simulink model "gm_HA_sys8_vnl"  (R2018a)
settings: Solver=FixedStepDiscrete  StartTime=0.0  StopTime=stopTime  RelTol=1e-3
InitFcn:
  | HA_sys8_init
StopFcn:
  | HA_sys8_freq_response
undefined symbols (not defined in the file or in its folder): dspDeleteFVToolLinkFromMask, FIRBandPass1, FIRBandPass2, FIRBandPass3, FIRBandPass4, FIRDecimator1, FIRDecimator2, FIRDecimator3, FIRDecimator4, FIRInterpolator1, FIRInterpolator2, FIRInterpolator3, FIRInterpolator4, Fs, Gain_B1_left, Gain_B1_right, Gain_B2_left, Gain_B2_right, Gain_B3_left, Gain_B3_right, Gain_B4_left, Gain_B4_right, Gain_left_all, Gain_right_all, gcbh
libraries: hdlsllib x40, dspmlti4 x32, simulink x4, dspsrcs4 x1
(part 1 of 4)
settings Model: Creator=The MathWorks, Inc.  LastModifiedBy=Ross_admin
settings DataIOCC: LimitDataPoints=on  SaveFormat=Array  SaveOutput=off  SaveTime=off
settings OptimizationCC: BlockReduction=off  ConditionallyExecuteInputs=off  DefaultParameterBehavior=Inlined  LifeSpan=inf
settings DebuggingCC: AlgebraicLoopMsg=error  InheritedTsInSrcMsg=none  SingleTaskRateTransMsg=error  AllowSymbolicDim=off  StrictBusMsg=ErrorOnBusTreatedAsVector  SFUnexpectedBacktrackingDiag=warning  SFNoUnconditionalDefaultTransitionDiag=warning  SFExecutionAtInitializationDiag=none
settings HardwareCC: ProdBitPerPointer=32  ProdBitPerSizeT=32  ProdBitPerPtrDiffT=32  ProdLargestAtomicFloat=None  ProdIntDivRoundTo=Undefined  ProdEndianess=Unspecified  ProdWordSize=32  ProdHWDeviceType=ASIC/FPGA->ASIC/FPGA  ProdEqTarget=off
settings ModelReferenceCC: PropagateSignalLabelsOutOfModel=off
settings CodeAppCC: StateflowObjectComments=on
settings GRTTargetCC: TargetLangStandard=C89/C90 (ANSI)  GeneratePreprocessorConditionals=Disable all
settings ConfigComp: CovMetricSettings=dw  CovHtmlReporting=on  CovSaveCumulativeToWorkspaceVar=on  CovSaveSingleToWorkspaceVar=on  CovShowResultsExplorer=off  CovExternalEMLEnable=off

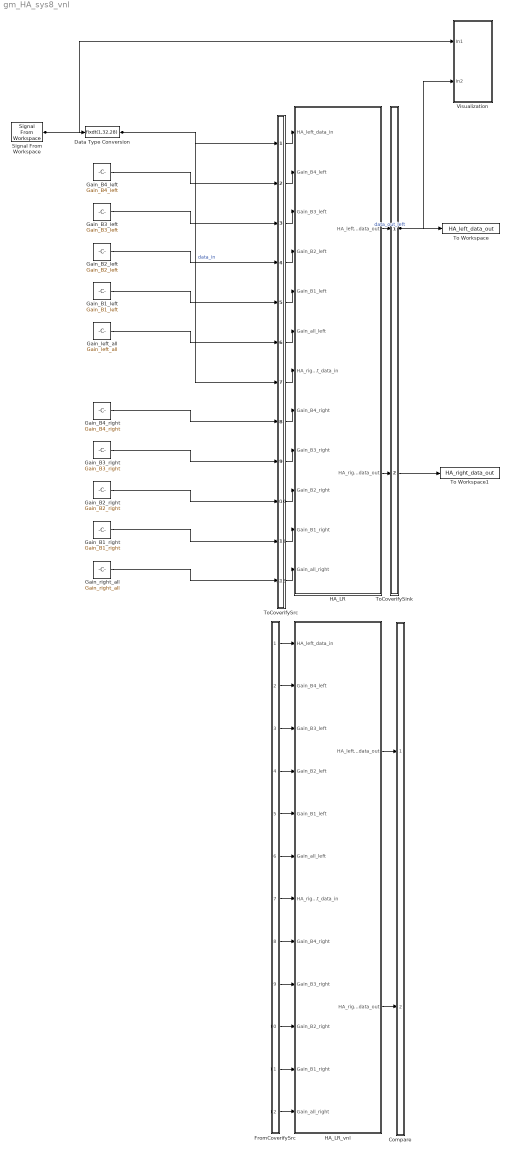
== system gm_HA_sys8_vnl ==
  Compare : Subsystem
      mask Display: disp('')
  Data Type Conversion : DataTypeConversion  OutDataTypeStr=fixdt(1,32,28)
  FromCoverifySrc : Subsystem
      mask Display: disp('')
  Gain_B1_left : Constant  Value=Gain_B1_left  OutDataTypeStr=fixdt(1,32,16)  SampleTime=-1  LockScale=on
  Gain_B1_right : Constant  Value=Gain_B1_right  OutDataTypeStr=fixdt(1,32,16)  SampleTime=-1  LockScale=on
  Gain_B2_left : Constant  Value=Gain_B2_left  OutDataTypeStr=fixdt(1,32,16)  SampleTime=-1  LockScale=on
  Gain_B2_right : Constant  Value=Gain_B2_right  OutDataTypeStr=fixdt(1,32,16)  SampleTime=-1  LockScale=on
  Gain_B3_left : Constant  Value=Gain_B3_left  OutDataTypeStr=fixdt(1,32,16)  SampleTime=-1  LockScale=on
  Gain_B3_right : Constant  Value=Gain_B3_right  OutDataTypeStr=fixdt(1,32,16)  SampleTime=-1  LockScale=on
  Gain_B4_left : Constant  Value=Gain_B4_left  OutDataTypeStr=fixdt(1,32,16)  SampleTime=-1  LockScale=on
  Gain_B4_right : Constant  Value=Gain_B4_right  OutDataTypeStr=fixdt(1,32,16)  SampleTime=-1  LockScale=on
  Gain_left_all : Constant  Value=Gain_left_all  OutDataTypeStr=fixdt(1,32,16)  SampleTime=-1  LockScale=on
  Gain_right_all : Constant  Value=Gain_right_all  OutDataTypeStr=fixdt(1,32,16)  SampleTime=-1  LockScale=on
  HA_LR : Subsystem
  HA_LR_vnl : Subsystem
  Signal From Workspace : dspsrcs4/Signal From Workspace  X=signal_in  Ts=1/Fs  nsamps=1  OutputAfterFinalValue=Setting to zero  ignoreOrWarnInputAndFrameLengths=off  OutputFrames=off
  To Workspace : ToWorkspace  VariableName=HA_left_data_out  SampleTime=-1
      settings: Save2DSignal=2-D array (concatenate along first dimension)
  To Workspace1 : ToWorkspace  VariableName=HA_right_data_out  SampleTime=-1
      settings: Save2DSignal=2-D array (concatenate along first dimension)
  ToCoverifySink : Subsystem
      mask Display: disp('')
  ToCoverifySrc : Subsystem
      mask Display: disp('')
  Visualization : Subsystem
      mask Display: disp('SCOPES')
  wires:
  Signal From Workspace/1 -> Visualization/1(In1), Data Type Conversion/1
  ToCoverifySrc/1(out1) -> HA_LR/1(HA_left_data_in)
  ToCoverifySrc/2(out2) -> HA_LR/2(Gain_B4_left)
  ToCoverifySrc/3(out3) -> HA_LR/3(Gain_B3_left)
  ToCoverifySrc/4(out4) -> HA_LR/4(Gain_B2_left)
  ToCoverifySrc/5(out5) -> HA_LR/5(Gain_B1_left)
  ToCoverifySrc/6(out6) -> HA_LR/6(Gain_all_left)
  ToCoverifySrc/7(out7) -> HA_LR/7(HA_right_data_in)
  ToCoverifySrc/8(out8) -> HA_LR/8(Gain_B4_right)
  ToCoverifySrc/9(out9) -> HA_LR/9(Gain_B3_right)
  ToCoverifySrc/10(out10) -> HA_LR/10(Gain_B2_right)
  ToCoverifySrc/11(out11) -> HA_LR/11(Gain_B1_right)
  ToCoverifySrc/12(out12) -> HA_LR/12(Gain_all_right)
  HA_LR/1(HA_left_data_out) -> ToCoverifySink/1(in1)  "data_out_left"
  HA_LR/2(HA_right_data_out) -> ToCoverifySink/2(in2)
  Data Type Conversion/1 -> ToCoverifySrc/1(in1), ToCoverifySrc/7(in7)  "data_in"
  Gain_B4_left/1 -> ToCoverifySrc/2(in2)
  Gain_B3_left/1 -> ToCoverifySrc/3(in3)
  Gain_B2_left/1 -> ToCoverifySrc/4(in4)
  Gain_B1_left/1 -> ToCoverifySrc/5(in5)
  Gain_left_all/1 -> ToCoverifySrc/6(in6)
  Gain_B4_right/1 -> ToCoverifySrc/8(in8)
  Gain_B3_right/1 -> ToCoverifySrc/9(in9)
  Gain_B2_right/1 -> ToCoverifySrc/10(in10)
  Gain_B1_right/1 -> ToCoverifySrc/11(in11)
  Gain_right_all/1 -> ToCoverifySrc/12(in12)
  ToCoverifySink/1(out1) -> To Workspace/1, Visualization/2(In2)
  ToCoverifySink/2(out2) -> To Workspace1/1
  FromCoverifySrc/1(out1) -> HA_LR_vnl/1(HA_left_data_in)
  FromCoverifySrc/2(out2) -> HA_LR_vnl/2(Gain_B4_left)
  FromCoverifySrc/3(out3) -> HA_LR_vnl/3(Gain_B3_left)
  FromCoverifySrc/4(out4) -> HA_LR_vnl/4(Gain_B2_left)
  FromCoverifySrc/5(out5) -> HA_LR_vnl/5(Gain_B1_left)
  FromCoverifySrc/6(out6) -> HA_LR_vnl/6(Gain_all_left)
  FromCoverifySrc/7(out7) -> HA_LR_vnl/7(HA_right_data_in)
  FromCoverifySrc/8(out8) -> HA_LR_vnl/8(Gain_B4_right)
  FromCoverifySrc/9(out9) -> HA_LR_vnl/9(Gain_B3_right)
  FromCoverifySrc/10(out10) -> HA_LR_vnl/10(Gain_B2_right)
  FromCoverifySrc/11(out11) -> HA_LR_vnl/11(Gain_B1_right)
  FromCoverifySrc/12(out12) -> HA_LR_vnl/12(Gain_all_right)
  HA_LR_vnl/1(HA_left_data_out) -> Compare/1(in1)
  HA_LR_vnl/2(HA_right_data_out) -> Compare/2(in2)

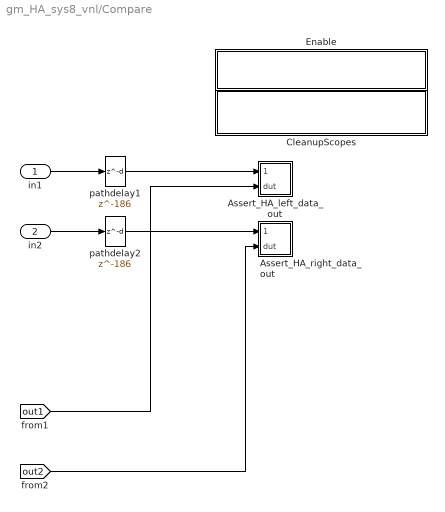
== system gm_HA_sys8_vnl/Compare ==
  in1 : Inport
  in2 : Inport  Port=2
  Assert_HA_left_data_out : Subsystem
  Assert_HA_right_data_out : Subsystem
  CleanupScopes : Subsystem
      settings: OpenFcn=|
      | blkName = gcb; %self block
      | idx = regexp(blkName, '/CleanupScopes$', 'once');
      | blkParent = blkName(1:idx-1);
      | blks=find_system(blkParent, 'LookUnderMasks', 'all','blocktype', 'Scope');
      | for itr = 1:length(blks)
      | 	 hScopeCfg = get_param(blks{itr},'ScopeConfiguration');
      | 	 hScopeCfg.Visible = ~ hScopeCfg.Visible;
      | end
      | drawnow;
      mask Display: fprintf(message('hdlcoder:cosim:vnl_dblclick').getString());
  Enable : Subsystem
      settings: OpenFcn=|
      | blkName = gcb;
      | idx = regexp(blkName, '/Enable$', 'once');
      | blkParent = blkName(1:idx-1);
      | blks=find_system(blkParent, 'LookUnderMasks', 'all','blocktype', 'Assertion');
      | e = get_param(blks{1}, 'Enabled');
      | if strcmp(e, 'on'), f= 'off';, else, f = 'on';, end
      | for ii=1:length(blks), set_param(blks{ii}, 'Enabled', f);, end
      | set_param(gcb, 'MaskDisplay',['fprintf(message(''hdlcoder:cosim:vnl_dblclick_assertions'',','''',upper(e),'''',').getString())']);
      mask Display: fprintf(message('hdlcoder:cosim:vnl_dblclick_assertions','OFF').getString());
  pathdelay1 : Delay  DelayLength=186
  pathdelay2 : Delay  DelayLength=186
  wires:
  in1/1 -> pathdelay1/1
  pathdelay1/1 -> Assert_HA_left_data_out/1(cosim)
  [out1] -> Assert_HA_left_data_out/2(dut)
  in2/1 -> pathdelay2/1
  pathdelay2/1 -> Assert_HA_right_data_out/1(cosim)
  [out2] -> Assert_HA_right_data_out/2(dut)

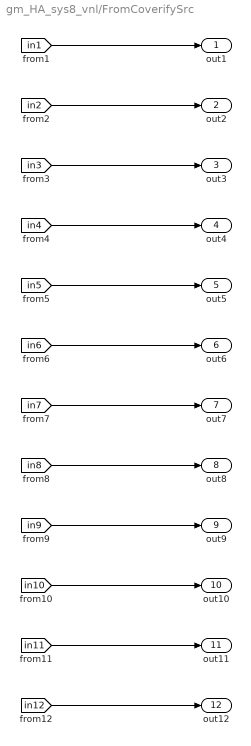
== system gm_HA_sys8_vnl/FromCoverifySrc ==
  out1 : Outport
  out2 : Outport  Port=2
  out3 : Outport  Port=3
  out4 : Outport  Port=4
  out5 : Outport  Port=5
  out6 : Outport  Port=6
  out7 : Outport  Port=7
  out8 : Outport  Port=8
  out9 : Outport  Port=9
  out10 : Outport  Port=10
  out11 : Outport  Port=11
  out12 : Outport  Port=12
  wires:
  [in1] -> out1/1
  [in2] -> out2/1
  [in3] -> out3/1
  [in4] -> out4/1
  [in5] -> out5/1
  [in6] -> out6/1
  [in7] -> out7/1
  [in8] -> out8/1
  [in9] -> out9/1
  [in10] -> out10/1
  [in11] -> out11/1
  [in12] -> out12/1

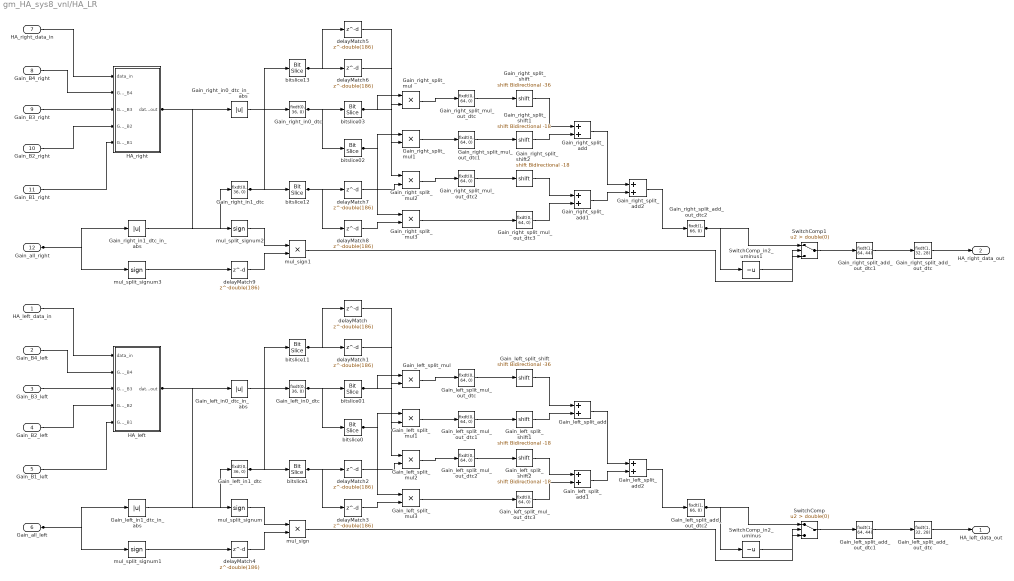
== system gm_HA_sys8_vnl/HA_LR ==
  HA_left_data_in : Inport  OutDataTypeStr=fixdt(1, 32, 28)  PortDimensions=1  SampleTime=2.08333333333333e-05
  Gain_B4_left : Inport  Port=2  OutDataTypeStr=fixdt(1, 32, 16)  PortDimensions=1  SampleTime=8.33333333333333e-05
  Gain_B3_left : Inport  Port=3  OutDataTypeStr=fixdt(1, 32, 16)  PortDimensions=1  SampleTime=0.000166666666666667
  Gain_B2_left : Inport  Port=4  OutDataTypeStr=fixdt(1, 32, 16)  PortDimensions=1  SampleTime=0.000333333333333333
  Gain_B1_left : Inport  Port=5  OutDataTypeStr=fixdt(1, 32, 16)  PortDimensions=1  SampleTime=0.000666666666666667
  Gain_all_left : Inport  Port=6  OutDataTypeStr=fixdt(1, 32, 16)  PortDimensions=1  SampleTime=2.08333333333333e-05
  HA_right_data_in : Inport  Port=7  OutDataTypeStr=fixdt(1, 32, 28)  PortDimensions=1  SampleTime=2.08333333333333e-05
  Gain_B4_right : Inport  Port=8  OutDataTypeStr=fixdt(1, 32, 16)  PortDimensions=1  SampleTime=8.33333333333333e-05
  Gain_B3_right : Inport  Port=9  OutDataTypeStr=fixdt(1, 32, 16)  PortDimensions=1  SampleTime=0.000166666666666667
  Gain_B2_right : Inport  Port=10  OutDataTypeStr=fixdt(1, 32, 16)  PortDimensions=1  SampleTime=0.000333333333333333
  Gain_B1_right : Inport  Port=11  OutDataTypeStr=fixdt(1, 32, 16)  PortDimensions=1  SampleTime=0.000666666666666667
  Gain_all_right : Inport  Port=12  OutDataTypeStr=fixdt(1, 32, 16)  PortDimensions=1  SampleTime=2.08333333333333e-05
  Gain_left_in0_dtc : DataTypeConversion  OutDataTypeStr=fixdt(0, 36, 0)  ConvertRealWorld=Stored Integer (SI)  SampleTime=2.08333333333333e-05
  Gain_left_in0_dtc_in_abs : Abs  SampleTime=2.08333333333333e-05  OutDataTypeStr=fixdt(0, 32, 28)
  Gain_left_in1_dtc : DataTypeConversion  OutDataTypeStr=fixdt(0, 36, 0)  ConvertRealWorld=Stored Integer (SI)  SampleTime=2.08333333333333e-05
  Gain_left_in1_dtc_in_abs : Abs  SampleTime=2.08333333333333e-05  OutDataTypeStr=fixdt(0, 32, 16)
  Gain_left_split_add : Sum  OutDataTypeStr=fixdt(0, 65, 0)  SampleTime=2.08333333333333e-05
  Gain_left_split_add1 : Sum  OutDataTypeStr=fixdt(0, 65, 0)  SampleTime=2.08333333333333e-05
  Gain_left_split_add2 : Sum  OutDataTypeStr=fixdt(0, 66, 0)  SampleTime=2.08333333333333e-05
  Gain_left_split_add_out_dtc : DataTypeConversion  OutDataTypeStr=fixdt(1, 32, 28)  SampleTime=2.08333333333333e-05  SaturateOnIntegerOverflow=on
  Gain_left_split_add_out_dtc1 : DataTypeConversion  OutDataTypeStr=fixdt(1, 64, 44)  ConvertRealWorld=Stored Integer (SI)  SampleTime=2.08333333333333e-05
  Gain_left_split_add_out_dtc2 : DataTypeConversion  OutDataTypeStr=fixdt(1, 66, 0)  SampleTime=2.08333333333333e-05
  Gain_left_split_mul : Product  Inputs=**  OutDataTypeStr=fixdt(0, 28, 0)  SampleTime=2.08333333333333e-05
  Gain_left_split_mul1 : Product  Inputs=**  OutDataTypeStr=uint32  SampleTime=2.08333333333333e-05
  Gain_left_split_mul2 : Product  Inputs=**  OutDataTypeStr=uint32  SampleTime=2.08333333333333e-05
  Gain_left_split_mul3 : Product  Inputs=**  OutDataTypeStr=fixdt(0, 36, 0)  SampleTime=2.08333333333333e-05
  Gain_left_split_mul_out_dtc{,1..3} (4 alike) : DataTypeConversion  OutDataTypeStr=fixdt(0, 64, 0)  SampleTime=2.08333333333333e-05
  Gain_left_split_shift : ArithShift  BitShiftNumber=-36
  Gain_left_split_shift1 : ArithShift  BitShiftNumber=-18
  Gain_left_split_shift2 : ArithShift  BitShiftNumber=-18
  Gain_right_in0_dtc : DataTypeConversion  OutDataTypeStr=fixdt(0, 36, 0)  ConvertRealWorld=Stored Integer (SI)  SampleTime=2.08333333333333e-05
  Gain_right_in0_dtc_in_abs : Abs  SampleTime=2.08333333333333e-05  OutDataTypeStr=fixdt(0, 32, 28)
  Gain_right_in1_dtc : DataTypeConversion  OutDataTypeStr=fixdt(0, 36, 0)  ConvertRealWorld=Stored Integer (SI)  SampleTime=2.08333333333333e-05
  Gain_right_in1_dtc_in_abs : Abs  SampleTime=2.08333333333333e-05  OutDataTypeStr=fixdt(0, 32, 16)
  Gain_right_split_add : Sum  OutDataTypeStr=fixdt(0, 65, 0)  SampleTime=2.08333333333333e-05
  Gain_right_split_add1 : Sum  OutDataTypeStr=fixdt(0, 65, 0)  SampleTime=2.08333333333333e-05
  Gain_right_split_add2 : Sum  OutDataTypeStr=fixdt(0, 66, 0)  SampleTime=2.08333333333333e-05
  Gain_right_split_add_out_dtc : DataTypeConversion  OutDataTypeStr=fixdt(1, 32, 28)  SampleTime=2.08333333333333e-05  SaturateOnIntegerOverflow=on
  Gain_right_split_add_out_dtc1 : DataTypeConversion  OutDataTypeStr=fixdt(1, 64, 44)  ConvertRealWorld=Stored Integer (SI)  SampleTime=2.08333333333333e-05
  Gain_right_split_add_out_dtc2 : DataTypeConversion  OutDataTypeStr=fixdt(1, 66, 0)  SampleTime=2.08333333333333e-05
  Gain_right_split_mul : Product  Inputs=**  OutDataTypeStr=fixdt(0, 28, 0)  SampleTime=2.08333333333333e-05
  Gain_right_split_mul1 : Product  Inputs=**  OutDataTypeStr=uint32  SampleTime=2.08333333333333e-05
  Gain_right_split_mul2 : Product  Inputs=**  OutDataTypeStr=uint32  SampleTime=2.08333333333333e-05
  Gain_right_split_mul3 : Product  Inputs=**  OutDataTypeStr=fixdt(0, 36, 0)  SampleTime=2.08333333333333e-05
  Gain_right_split_mul_out_dtc{,1..3} (4 alike) : DataTypeConversion  OutDataTypeStr=fixdt(0, 64, 0)  SampleTime=2.08333333333333e-05
  Gain_right_split_shift : ArithShift  BitShiftNumber=-36
  Gain_right_split_shift1 : ArithShift  BitShiftNumber=-18
  Gain_right_split_shift2 : ArithShift  BitShiftNumber=-18
  HA_left : Subsystem
  HA_right : Subsystem
  SwitchComp : Switch  Criteria=u2 > Threshold  Threshold=double(0)  OutDataTypeStr=fixdt(1, 66, 0)  SampleTime=2.08333333333333e-05
  SwitchComp1 : Switch  Criteria=u2 > Threshold  Threshold=double(0)  OutDataTypeStr=fixdt(1, 66, 0)  SampleTime=2.08333333333333e-05
  SwitchComp_in2_uminus : UnaryMinus  SampleTime=2.08333333333333e-05
  SwitchComp_in2_uminus1 : UnaryMinus  SampleTime=2.08333333333333e-05
  bitslice0 : hdlsllib/Logic and Bit Operations/Bit Slice  lidx=double(17)  ridx=double(0)
  bitslice01 : hdlsllib/Logic and Bit Operations/Bit Slice  lidx=double(31)  ridx=double(18)
  bitslice02 : hdlsllib/Logic and Bit Operations/Bit Slice  lidx=double(17)  ridx=double(0)
  bitslice03 : hdlsllib/Logic and Bit Operations/Bit Slice  lidx=double(31)  ridx=double(18)
  bitslice1 : hdlsllib/Logic and Bit Operations/Bit Slice  lidx=double(17)  ridx=double(0)
  bitslice11 : hdlsllib/Logic and Bit Operations/Bit Slice  lidx=double(31)  ridx=double(18)
  bitslice12 : hdlsllib/Logic and Bit Operations/Bit Slice  lidx=double(17)  ridx=double(0)
  bitslice13 : hdlsllib/Logic and Bit Operations/Bit Slice  lidx=double(31)  ridx=double(18)
  delayMatch{,1..9} (10 alike) : Delay  DelayLength=double(186)  InitialCondition=0  InputProcessing=Inherited  SampleTime=2.08333333333333e-05
  mul_sign : Product  Inputs=**  OutDataTypeStr=fixdt(1, 2, 0)  SampleTime=2.08333333333333e-05
  mul_sign1 : Product  Inputs=**  OutDataTypeStr=fixdt(1, 2, 0)  SampleTime=2.08333333333333e-05
  mul_split_signum{,1..3} (4 alike) : Signum  SampleTime=2.08333333333333e-05
  HA_left_data_out : Outport
  HA_right_data_out : Outport  Port=2
  wires:
  mul_split_signum3/1 -> delayMatch9/1
  bitslice12/1 -> delayMatch7/1, delayMatch8/1
  delayMatch8/1 -> Gain_right_split_mul3/2
  bitslice13/1 -> delayMatch5/1, delayMatch6/1
  delayMatch6/1 -> Gain_right_split_mul1/2
  mul_split_signum1/1 -> delayMatch4/1
  bitslice1/1 -> delayMatch2/1, delayMatch3/1
  delayMatch3/1 -> Gain_left_split_mul3/2
  bitslice11/1 -> delayMatch/1, delayMatch1/1
  delayMatch1/1 -> Gain_left_split_mul1/2
  SwitchComp_in2_uminus1/1 -> SwitchComp1/3
  SwitchComp1/1 -> Gain_right_split_add_out_dtc1/1
  Gain_right_split_add2/1 -> Gain_right_split_add_out_dtc2/1
  mul_sign1/1 -> SwitchComp1/2
  delayMatch9/1 -> mul_sign1/2
  Gain_right_in1_dtc_in_abs/1 -> Gain_right_in1_dtc/1
  mul_split_signum2/1 -> mul_sign1/1
  Gain_right_in0_dtc_in_abs/1 -> Gain_right_in0_dtc/1
  Gain_right_split_add_out_dtc2/1 -> SwitchComp1/1, SwitchComp_in2_uminus1/1
  Gain_right_split_add_out_dtc1/1 -> Gain_right_split_add_out_dtc/1
  Gain_right_split_add_out_dtc/1 -> HA_right_data_out/1
  Gain_right_split_add1/1 -> Gain_right_split_add2/2
  Gain_right_split_add/1 -> Gain_right_split_add2/1
  Gain_right_split_mul3/1 -> Gain_right_split_mul_out_dtc3/1
  Gain_right_split_mul_out_dtc3/1 -> Gain_right_split_add1/2
  Gain_right_split_shift2/1 -> Gain_right_split_add1/1
  Gain_right_split_mul2/1 -> Gain_right_split_mul_out_dtc2/1
  Gain_right_split_mul_out_dtc2/1 -> Gain_right_split_shift2/1
  Gain_right_split_shift1/1 -> Gain_right_split_add/2
  Gain_right_split_mul1/1 -> Gain_right_split_mul_out_dtc1/1
  Gain_right_split_mul_out_dtc1/1 -> Gain_right_split_shift1/1
  Gain_right_split_shift/1 -> Gain_right_split_add/1
  Gain_right_split_mul/1 -> Gain_right_split_mul_out_dtc/1
  Gain_right_split_mul_out_dtc/1 -> Gain_right_split_shift/1
  delayMatch5/1 -> Gain_right_split_mul/2
  delayMatch7/1 -> Gain_right_split_mul2/2
  bitslice03/1 -> Gain_right_split_mul/1, Gain_right_split_mul2/1
  bitslice02/1 -> Gain_right_split_mul1/1, Gain_right_split_mul3/1
  Gain_right_in1_dtc/1 -> bitslice12/1, bitslice13/1
  Gain_right_in0_dtc/1 -> bitslice02/1, bitslice03/1
  SwitchComp_in2_uminus/1 -> SwitchComp/3
  SwitchComp/1 -> Gain_left_split_add_out_dtc1/1
  Gain_left_split_add2/1 -> Gain_left_split_add_out_dtc2/1
  mul_sign/1 -> SwitchComp/2
  delayMatch4/1 -> mul_sign/2
  Gain_left_in1_dtc_in_abs/1 -> Gain_left_in1_dtc/1
  mul_split_signum/1 -> mul_sign/1
  Gain_left_in0_dtc_in_abs/1 -> Gain_left_in0_dtc/1
  Gain_left_split_add_out_dtc2/1 -> SwitchComp/1, SwitchComp_in2_uminus/1
  Gain_left_split_add_out_dtc1/1 -> Gain_left_split_add_out_dtc/1
  Gain_left_split_add_out_dtc/1 -> HA_left_data_out/1
  Gain_left_split_add1/1 -> Gain_left_split_add2/2
  Gain_left_split_add/1 -> Gain_left_split_add2/1
  Gain_left_split_mul3/1 -> Gain_left_split_mul_out_dtc3/1
  Gain_left_split_mul_out_dtc3/1 -> Gain_left_split_add1/2
  Gain_left_split_shift2/1 -> Gain_left_split_add1/1
  Gain_left_split_mul2/1 -> Gain_left_split_mul_out_dtc2/1
  Gain_left_split_mul_out_dtc2/1 -> Gain_left_split_shift2/1
  Gain_left_split_shift1/1 -> Gain_left_split_add/2
  Gain_left_split_mul1/1 -> Gain_left_split_mul_out_dtc1/1
  Gain_left_split_mul_out_dtc1/1 -> Gain_left_split_shift1/1
  Gain_left_split_shift/1 -> Gain_left_split_add/1
  Gain_left_split_mul/1 -> Gain_left_split_mul_out_dtc/1
  Gain_left_split_mul_out_dtc/1 -> Gain_left_split_shift/1
  delayMatch/1 -> Gain_left_split_mul/2
  delayMatch2/1 -> Gain_left_split_mul2/2
  bitslice01/1 -> Gain_left_split_mul/1, Gain_left_split_mul2/1
  bitslice0/1 -> Gain_left_split_mul1/1, Gain_left_split_mul3/1
  Gain_left_in1_dtc/1 -> bitslice1/1, bitslice11/1
  Gain_left_in0_dtc/1 -> bitslice0/1, bitslice01/1
  HA_right/1(data_out) -> Gain_right_in0_dtc_in_abs/1, mul_split_signum2/1
  HA_left/1(data_out) -> Gain_left_in0_dtc_in_abs/1, mul_split_signum/1
  Gain_all_right/1 -> Gain_right_in1_dtc_in_abs/1, mul_split_signum3/1
  Gain_B1_right/1 -> HA_right/5(Gain_B1)
  Gain_B2_right/1 -> HA_right/4(Gain_B2)
  Gain_B3_right/1 -> HA_right/3(Gain_B3)
  Gain_B4_right/1 -> HA_right/2(Gain_B4)
  HA_right_data_in/1 -> HA_right/1(data_in)
  Gain_all_left/1 -> Gain_left_in1_dtc_in_abs/1, mul_split_signum1/1
  Gain_B1_left/1 -> HA_left/5(Gain_B1)
  Gain_B2_left/1 -> HA_left/4(Gain_B2)
  Gain_B3_left/1 -> HA_left/3(Gain_B3)
  Gain_B4_left/1 -> HA_left/2(Gain_B4)
  HA_left_data_in/1 -> HA_left/1(data_in)

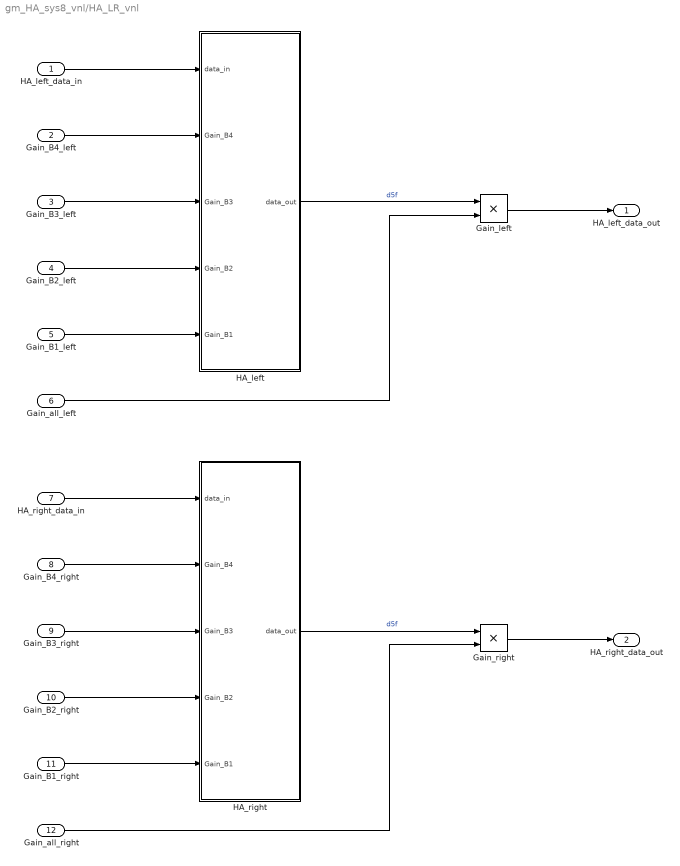
== system gm_HA_sys8_vnl/HA_LR_vnl ==
  HA_left_data_in : Inport
  Gain_B4_left : Inport  Port=2
  Gain_B3_left : Inport  Port=3
  Gain_B2_left : Inport  Port=4
  Gain_B1_left : Inport  Port=5
  Gain_all_left : Inport  Port=6
  HA_right_data_in : Inport  Port=7
  Gain_B4_right : Inport  Port=8
  Gain_B3_right : Inport  Port=9
  Gain_B2_right : Inport  Port=10
  Gain_B1_right : Inport  Port=11
  Gain_all_right : Inport  Port=12
  Gain_left : Product  OutDataTypeStr=fixdt(1,32,28)  SaturateOnIntegerOverflow=on
  Gain_right : Product  OutDataTypeStr=fixdt(1,32,28)  SaturateOnIntegerOverflow=on
  HA_left : Subsystem
  HA_right : Subsystem
  HA_left_data_out : Outport
  HA_right_data_out : Outport  Port=2
  wires:
  HA_right/1(data_out) -> Gain_right/1  "d5f"
  Gain_all_right/1 -> Gain_right/2
  HA_right_data_in/1 -> HA_right/1(data_in)
  Gain_B3_right/1 -> HA_right/3(Gain_B3)
  Gain_B2_right/1 -> HA_right/4(Gain_B2)
  Gain_right/1 -> HA_right_data_out/1
  Gain_B4_right/1 -> HA_right/2(Gain_B4)
  Gain_B1_right/1 -> HA_right/5(Gain_B1)
  Gain_left/1 -> HA_left_data_out/1
  Gain_all_left/1 -> Gain_left/2
  HA_left/1(data_out) -> Gain_left/1  "d5f"
  Gain_B4_left/1 -> HA_left/2(Gain_B4)
  HA_left_data_in/1 -> HA_left/1(data_in)
  Gain_B2_left/1 -> HA_left/4(Gain_B2)
  Gain_B3_left/1 -> HA_left/3(Gain_B3)
  Gain_B1_left/1 -> HA_left/5(Gain_B1)

== system gm_HA_sys8_vnl/ToCoverifySink ==
  in1 : Inport
  in2 : Inport  Port=2
  out1 : Outport
  out2 : Outport  Port=2
  tag scope: out1=global, out2=global
  wires:
  in1/1 -> out1/1, [out1]
  in2/1 -> out2/1, [out2]

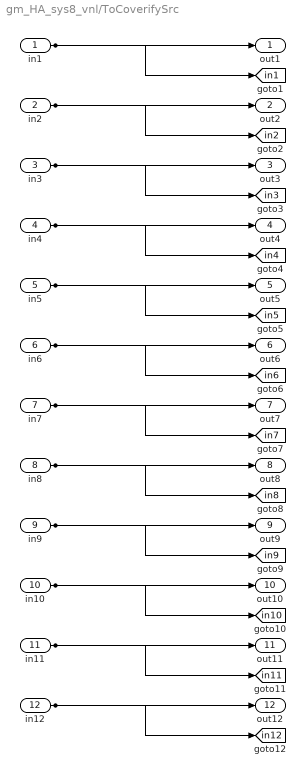
== system gm_HA_sys8_vnl/ToCoverifySrc ==
  in1 : Inport
  in2 : Inport  Port=2
  in3 : Inport  Port=3
  in4 : Inport  Port=4
  in5 : Inport  Port=5
  in6 : Inport  Port=6
  in7 : Inport  Port=7
  in8 : Inport  Port=8
  in9 : Inport  Port=9
  in10 : Inport  Port=10
  in11 : Inport  Port=11
  in12 : Inport  Port=12
  out1 : Outport
  out2 : Outport  Port=2
  out3 : Outport  Port=3
  out4 : Outport  Port=4
  out5 : Outport  Port=5
  out6 : Outport  Port=6
  out7 : Outport  Port=7
  out8 : Outport  Port=8
  out9 : Outport  Port=9
  out10 : Outport  Port=10
  out11 : Outport  Port=11
  out12 : Outport  Port=12
  tag scope: in10=global, in11=global, in12=global, in1=global, in2=global, in3=global, in4=global, in5=global, in6=global, in7=global, in8=global, in9=global
  wires:
  in1/1 -> out1/1, [in1]
  in2/1 -> out2/1, [in2]
  in3/1 -> out3/1, [in3]
  in4/1 -> out4/1, [in4]
  in5/1 -> out5/1, [in5]
  in6/1 -> out6/1, [in6]
  in7/1 -> out7/1, [in7]
  in8/1 -> out8/1, [in8]
  in9/1 -> out9/1, [in9]
  in10/1 -> out10/1, [in10]
  in11/1 -> out11/1, [in11]
  in12/1 -> out12/1, [in12]

== system gm_HA_sys8_vnl/Visualization ==
  In1 : Inport
  In2 : Inport  Port=2
  Input Signal (dB Magnitude) : Scope
  Input Signal Spectrum : SpectrumAnalyzer
  Output Signal (dB Mag - passband scale) : Scope
  Output Signal Spectrum : SpectrumAnalyzer
  wires:
  In1/1 -> Input Signal Spectrum/1, Input Signal (dB Magnitude)/1
  In2/1 -> Output Signal Spectrum/1, Output Signal (dB Mag - passband scale)/1

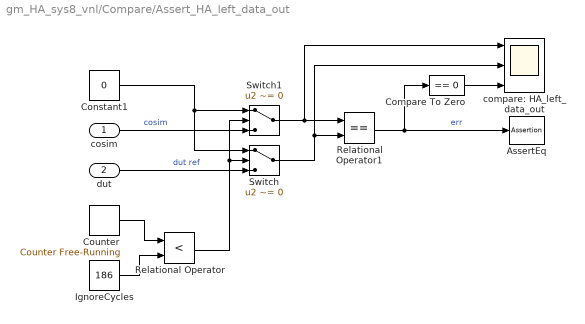
== system gm_HA_sys8_vnl/Compare/Assert_HA_left_data_out ==
  cosim : Inport
  dut : Inport  Port=2
  AssertEq : Assertion  StopWhenAssertionFail=off
  Compare To Zero : simulink/Logic and Bit Operations/Compare To Zero  relop===  OutDataTypeStr=boolean
  Constant1 : Constant  Value=0  OutDataTypeStr=Inherit: Inherit via back propagation  SampleTime=-1
  Counter : simulink/Sources/Counter Free-Running  NumBits=32  tsamp=-1
  IgnoreCycles : Constant  Value=186  OutDataTypeStr=Inherit: Inherit via back propagation  SampleTime=-1
  Relational Operator : RelationalOperator  Operator=<  OutDataTypeStr=boolean  RndMeth=Nearest
  Relational Operator1 : RelationalOperator  Operator===  OutDataTypeStr=boolean  RndMeth=Nearest
  Switch : Switch  Criteria=u2 ~= 0
  Switch1 : Switch  Criteria=u2 ~= 0
  compare: HA_left_data_out : Scope  NumInputPorts=3
  wires:
  Compare To Zero/1 -> compare: HA_left_data_out/3
  Relational Operator1/1 -> Compare To Zero/1, AssertEq/1  "err"
  Switch1/1 -> compare: HA_left_data_out/1, Relational Operator1/1
  Switch/1 -> compare: HA_left_data_out/2, Relational Operator1/2
  Constant1/1 -> Switch/1, Switch1/1
  Relational Operator/1 -> Switch/2, Switch1/2
  cosim/1 -> Switch1/3  "cosim"
  dut/1 -> Switch/3  "dut ref"
  Counter/1 -> Relational Operator/1
  IgnoreCycles/1 -> Relational Operator/2

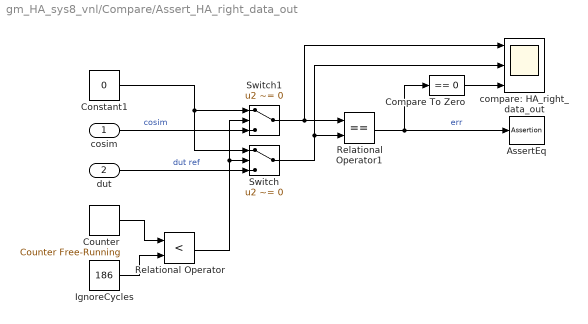
== system gm_HA_sys8_vnl/Compare/Assert_HA_right_data_out ==
  cosim : Inport
  dut : Inport  Port=2
  AssertEq : Assertion  StopWhenAssertionFail=off
  Compare To Zero : simulink/Logic and Bit Operations/Compare To Zero  relop===  OutDataTypeStr=boolean
  Constant1 : Constant  Value=0  OutDataTypeStr=Inherit: Inherit via back propagation  SampleTime=-1
  Counter : simulink/Sources/Counter Free-Running  NumBits=32  tsamp=-1
  IgnoreCycles : Constant  Value=186  OutDataTypeStr=Inherit: Inherit via back propagation  SampleTime=-1
  Relational Operator : RelationalOperator  Operator=<  OutDataTypeStr=boolean  RndMeth=Nearest
  Relational Operator1 : RelationalOperator  Operator===  OutDataTypeStr=boolean  RndMeth=Nearest
  Switch : Switch  Criteria=u2 ~= 0
  Switch1 : Switch  Criteria=u2 ~= 0
  compare: HA_right_data_out : Scope  NumInputPorts=3
  wires:
  Compare To Zero/1 -> compare: HA_right_data_out/3
  Relational Operator1/1 -> Compare To Zero/1, AssertEq/1  "err"
  Switch1/1 -> compare: HA_right_data_out/1, Relational Operator1/1
  Switch/1 -> compare: HA_right_data_out/2, Relational Operator1/2
  Constant1/1 -> Switch/1, Switch1/1
  Relational Operator/1 -> Switch/2, Switch1/2
  cosim/1 -> Switch1/3  "cosim"
  dut/1 -> Switch/3  "dut ref"
  Counter/1 -> Relational Operator/1
  IgnoreCycles/1 -> Relational Operator/2

== system gm_HA_sys8_vnl/Compare/CleanupScopes ==

== system gm_HA_sys8_vnl/Compare/Enable ==
